simulink model "OLD_of_Vehicle_model_testing"  (R2016b)
settings: Solver=ode3  StartTime=0.0  StopTime=50  RelTol=1e-3
settings Model: Creator=liana  LastModifiedBy=liana

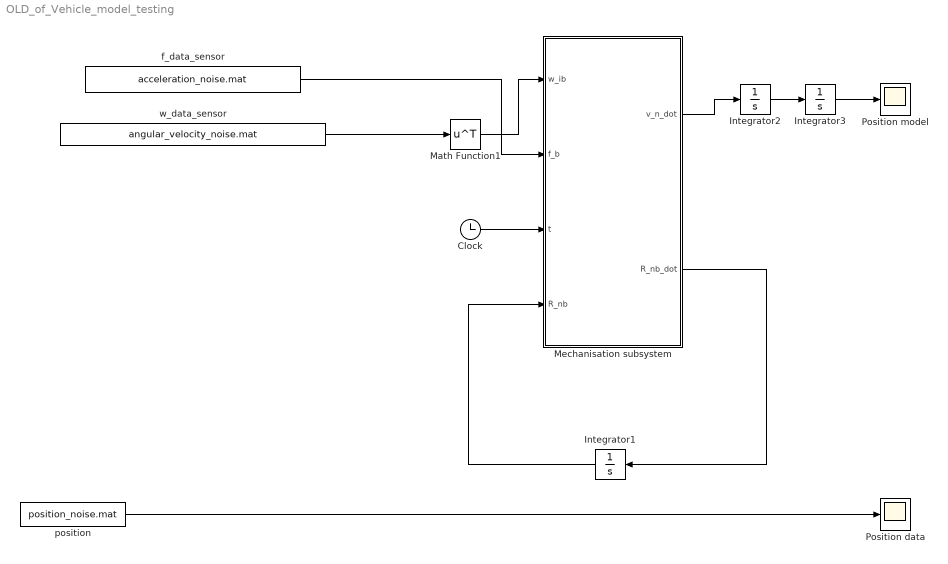
== system OLD_of_Vehicle_model_testing ==
  Clock : Clock
  Integrator1 : Integrator
  Integrator2 : Integrator
  Integrator3 : Integrator
  Math Function1 : Math  Operator=transpose  SaturateOnIntegerOverflow=on
  Mechanisation subsystem : Subsystem
  Position data : Scope
  Position model : Scope
  f_data_sensor : FromFile  FileName=acceleration_noise.mat  SampleTime=0
  position : FromFile  FileName=position_noise.mat  SampleTime=0
  w_data_sensor : FromFile  FileName=angular_velocity_noise.mat  SampleTime=0
  wires:
  w_data_sensor/1 -> Math Function1/1
  Mechanisation subsystem/1(v_n_dot) -> Integrator2/1
  Integrator2/1 -> Integrator3/1
  Math Function1/1 -> Mechanisation subsystem/1(w_ib)
  Clock/1 -> Mechanisation subsystem/3(t)
  position/1 -> Position data/1
  f_data_sensor/1 -> Mechanisation subsystem/2(f_b)
  Integrator3/1 -> Position model/1
  Mechanisation subsystem/2(R_nb_dot) -> Integrator1/1
  Integrator1/1 -> Mechanisation subsystem/4("R_nb ")

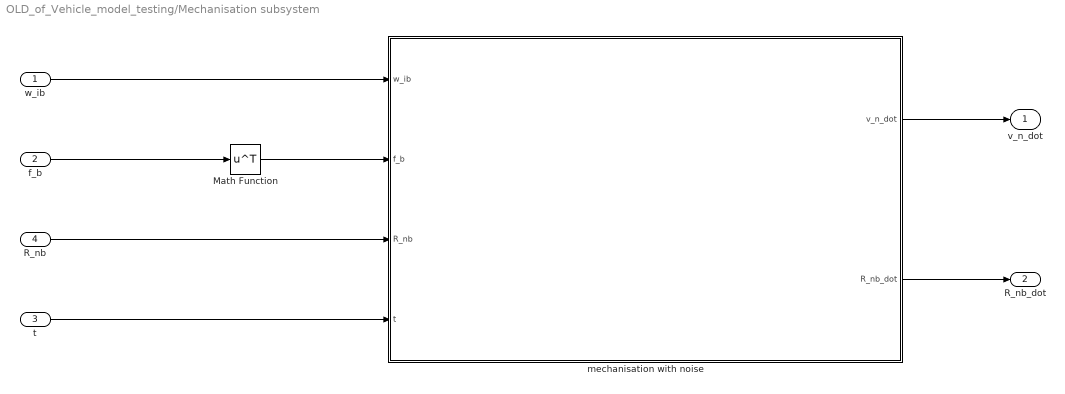
== system OLD_of_Vehicle_model_testing/Mechanisation subsystem ==
  w_ib : Inport
  f_b : Inport  Port=2
  t : Inport  Port=3
  "R_nb " : Inport  Port=4
  Math Function : Math  Operator=transpose  SaturateOnIntegerOverflow=on
  mechanisation with noise : MATLAB Function  TreatAsAtomicUnit=on
  v_n_dot : Outport
  R_nb_dot : Outport  Port=2
  wires:
  t/1 -> mechanisation with noise/4(t)
  f_b/1 -> Math Function/1
  mechanisation with noise/1(v_n_dot) -> v_n_dot/1
  mechanisation with noise/2(R_nb_dot) -> R_nb_dot/1
  "R_nb "/1 -> mechanisation with noise/3(R_nb)
  Math Function/1 -> mechanisation with noise/2(f_b)
  w_ib/1 -> mechanisation with noise/1(w_ib)

== matlab function OLD_of_Vehicle_model_testing/Mechanisation subsystem/mechanisation with noise ==
  data: w_ib input; f_b input; v_n_dot output; R_nb_dot output; R_nb input; t input
function [v_n_dot, R_nb_dot] = mechanisation(w_ib, f_b, R_nb, t)



g_n = [0 0 -9.8]';

% w_ib = size(3,1);

if t == 0
    v_n_dot = zeros(3,1);
    R_nb_dot = eye(3);
    R_nb = eye(3);
end

Skew = skew(w_ib);


%p_dot = v_n;

v_n_dot = R_nb * f_b + g_n;

R_nb_dot = R_nb * Skew;
